simulink model "SPPMSM_DynoLoadTorque_sfun"  (R2022b)
settings: Solver=FixedStepDiscrete  StartTime=0.0  StopTime=SimTime  FixedStep=Ts_Model  RelTol=1e-3
undefined symbols (not defined in the file): theta_m_0
libraries: MapleSim_v142IE_1000 x1, MapleSim_v142IE_200 x1, MapleSim_v142IE_400 x1
settings Model: Creator=BEDNASA  LastModifiedBy=HENRIE2
settings SolverCC: AlgebraicLoopSolver=TrustRegion
settings DebuggingCC: UnconnectedInputMsg=warning  UnconnectedOutputMsg=warning  UnconnectedLineMsg=warning  SFMachineParentedDataDiag=warning
settings ModelReferenceCC: EnableRefExpFcnMdlSchedulingChecks=on
settings RTWCC: CustomInclude="\"C:\\Users\\BEDNASA\\Desktop\\SPPMSM\\SPPMSM\\SinglePhaseSimArch_alpha\\tools\\FMIKit-Simulink-2.8\\include\" \"C:\\Users\\BEDNASA\\Desktop\\VA_PSCSimulationArchitecture (2)\\VA_PSCSimulationArchitecture\\tools\\FMIKit-Simulink-2.7\\include\" \"C:\\Users\\BEDNASA\\Desktop\\SPPMSM\\SPPMSM\\MBD_SPM_SimArch\\tools\\include\" \"C:\\Users\\BEDNASA\\Desktop\\SPPMSM\\SPPMSM\\MBD_SPM_SimArch\\tools\\FMIKit\\FMIKit-Simulink-2.9\\include\" \"C:\\Data\\MBD_SPM_SimArch\\tools\\FMIKit\\FMIKit-Simulink-2.9\\include\" \"C:\\Users\\BEDNASA\\Desktop\\Projects\\MBD_SPM_SimArch_v02beta\\MBD_SPM_SimArch\\tools\\FMIKit\\FMIKit-Simulink-2.9\\include\" \"C:\\Data\\Szymon_Projects\\MBD_SPM_SimArch\\tools\\FMIKit\\FMIKit-Simulink-2.9\\include\" \"C:\\Data\\MBD_SPM_SimArch_TEST3\\tools\\FMIKit\\FMIKit-Simulink-2.9\\include\""  CustomSource="\"C:\\Users\\BEDNASA\\Desktop\\SPPMSM\\SPPMSM\\SinglePhaseSimArch_alpha\\tools\\FMIKit-Simulink-2.8\\src\\FMU.cpp\" \"C:\\Users\\BEDNASA\\Desktop\\SPPMSM\\SPPMSM\\SinglePhaseSimArch_alpha\\tools\\FMIKit-Simulink-2.8\\src\\FMU1.cpp\" \"C:\\Users\\BEDNASA\\Desktop\\SPPMSM\\SPPMSM\\SinglePhaseSimArch_alpha\\tools\\FMIKit-Simulink-2.8\\src\\FMU2.cpp\" \"C:\\Users\\BEDNASA\\Desktop\\VA_PSCSimulationArchitecture (2)\\VA_PSCSimulationArchitecture\\tools\\FMIKit-Simulink-2.7\\src\\FMU.cpp\" \"C:\\Users\\BEDNASA\\Desktop\\VA_PSCSimulationArchitecture (2)\\VA_PSCSimulationArchitecture\\tools\\FMIKit-Simulink-2.7\\src\\FMU1.cpp\" \"C:\\Users\\BEDNASA\\Desktop\\VA_PSCSimulationArchitecture (2)\\VA_PSCSimulationArchitecture\\tools\\FMIKit-Simulink-2.7\\src\\FMU2.cpp\" \"C:\\Users\\BEDNASA\\Desktop\\SPPMSM\\SPPMSM\\MBD_SPM_SimArch\\tools\\src\\FMU.cpp\" \"C:\\Users\\BEDNASA\\Desktop\\SPPMSM\\SPPMSM\\MBD_SPM_SimArch\\tools\\src\\FMU1.cpp\" \"C:\\Users\\BEDNASA\\Desktop\\SPPMSM\\SPPMSM\\MBD_SPM_SimArch\\tools\\src\\FMU2.cpp\" \"C:\\Users\\BEDNASA\\Desktop\\SPPMSM\\SPPMSM\\MBD_SPM_SimArch\\tools\\FMIKit\\FMIKit-Simulink-2.9\\src\\FMU.cpp\" \"C:\\Users\\BEDNASA\\Desktop\\SPPMSM\\SPPMSM\\MBD_SPM_SimArch\\tools\\FMIKit\\FMIKit-Simulink-2.9\\src\\FMU1.cpp\" \"C:\\Users\\BEDNASA\\Desktop\\SPPMSM\\SPPMSM\\MBD_SPM_SimArch\\tools\\FMIKit\\FMIKit-Simulink-2.9\\src\\FMU2.cpp\" \"C:\\Data\\MBD_SPM_SimArch\\tools\\FMIKit\\FMIKit-Simulink-2.9\\src\\FMU.cpp\" \"C:\\Data\\MBD_SPM_SimArch\\tools\\FMIKit\\FMIKit-Simulink-2.9\\src\\FMU1.cpp\" \"C:\\Data\\MBD_SPM_SimArch\\tools\\FMIKit\\FMIKit-Simulink-2.9\\src\\FMU2.cpp\" \"C:\\Users\\BEDNASA\\Desktop\\Projects\\MBD_SPM_SimArch_v02beta\\MBD_SPM_SimArch\\tools\\FMIKit\\FMIKit-Simulink-2.9\\src\\FMU.cpp\" \"C:\\Users\\BEDNASA\\Desktop\\Projects\\MBD_SPM_SimArch_v02beta\\MBD_SPM_SimArch\\tools\\FMIKit\\FMIKit-Simulink-2.9\\src\\FMU1.cpp\" \"C:\\Users\\BEDNASA\\Desktop\\Projects\\MBD_SPM_SimArch_v02beta\\MBD_SPM_SimArch\\tools\\FMIKit\\FMIKit-Simulink-2.9\\src\\FMU2.cpp\" \"C:\\Data\\Szymon_Projects\\MBD_SPM_SimArch\\tools\\FMIKit\\FMIKit-Simulink-2.9\\src\\FMU.cpp\" \"C:\\Data\\Szymon_Projects\\MBD_SPM_SimArch\\tools\\FMIKit\\FMIKit-Simulink-2.9\\src\\FMU1.cpp\" \"C:\\Data\\Szymon_Projects\\MBD_SPM_SimArch\\tools\\FMIKit\\FMIKit-Simulink-2.9\\src\\FMU2.cpp\" \"C:\\Data\\MBD_SPM_SimArch_TEST3\\tools\\FMIKit\\FMIKit-Simulink-2.9\\src\\FMU.cpp\" \"C:\\Data\\MBD_SPM_SimArch_TEST3\\tools\\FMIKit\\FMIKit-Simulink-2.9\\src\\FMU1.cpp\" \"C:\\Data\\MBD_SPM_SimArch_TEST3\\tools\\FMIKit\\FMIKit-Simulink-2.9\\src\\FMU2.cpp\""  CustomLibrary="\"C:\\Program Files\\Microsoft SDKs\\Windows\\v6.0A\\Lib\\x64\\ShLwApi.Lib\""

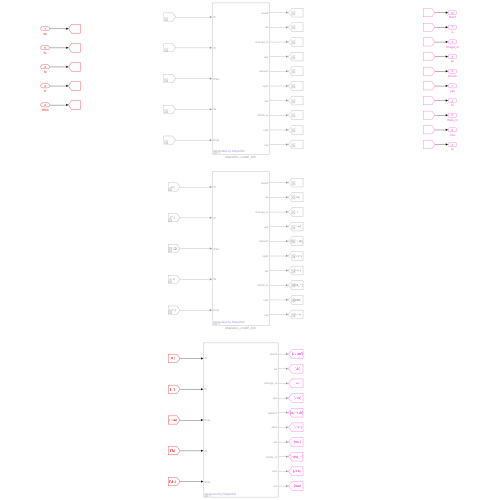
[thumbnail: Simulink's stored preview of the top-level diagram]
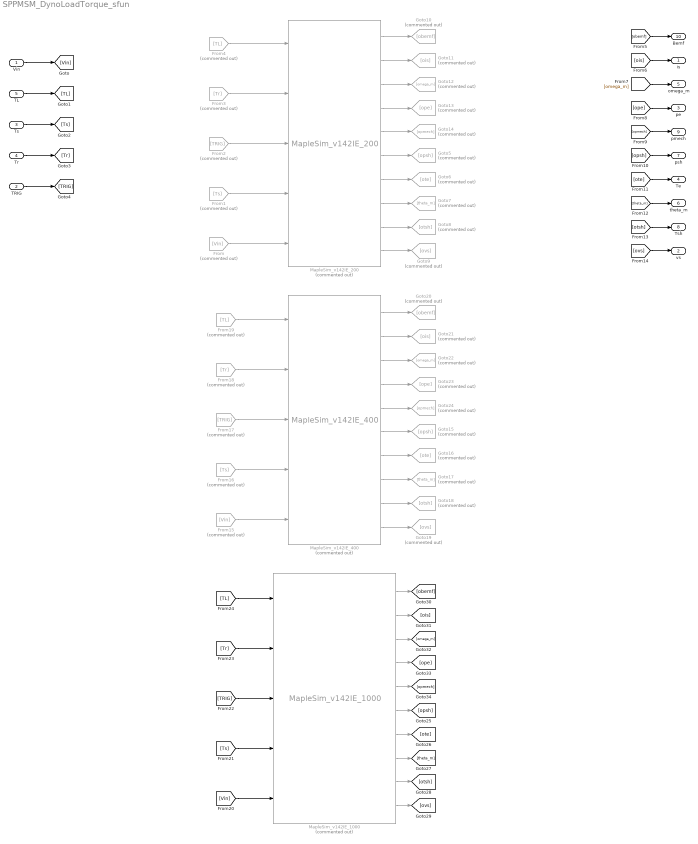
== system SPPMSM_DynoLoadTorque_sfun ==
  Vin : Inport
  TRIG : Inport  Port=2
  Ts : Inport  Port=3
  Tr : Inport  Port=4
  TL : Inport  Port=5
  From : From  Commented=on  GotoTag=Vin
  From1 : From  Commented=on  GotoTag=Ts
  From15 : From  Commented=on  GotoTag=Vin
  From16 : From  Commented=on  GotoTag=Ts
  From17 : From  Commented=on  GotoTag=TRIG
  From18 : From  Commented=on  GotoTag=Tr
  From19 : From  Commented=on  GotoTag=TL
  From2 : From  Commented=on  GotoTag=TRIG
  From3 : From  Commented=on  GotoTag=Tr
  From4 : From  Commented=on  GotoTag=TL
  Goto10 : Goto  Commented=on  GotoTag=obemf
  Goto11 : Goto  Commented=on  GotoTag=ois
  Goto12 : Goto  Commented=on  GotoTag=omega_m
  Goto13 : Goto  Commented=on  GotoTag=ope
  Goto14 : Goto  Commented=on  GotoTag=opmech
  Goto15 : Goto  Commented=on  GotoTag=opsh
  Goto16 : Goto  Commented=on  GotoTag=ote
  Goto17 : Goto  Commented=on  GotoTag=theta_m
  Goto18 : Goto  Commented=on  GotoTag=otsh
  Goto19 : Goto  Commented=on  GotoTag=ovs
  Goto20 : Goto  Commented=on  GotoTag=obemf
  Goto21 : Goto  Commented=on  GotoTag=ois
  Goto22 : Goto  Commented=on  GotoTag=omega_m
  Goto23 : Goto  Commented=on  GotoTag=ope
  Goto24 : Goto  Commented=on  GotoTag=opmech
  Goto5 : Goto  Commented=on  GotoTag=opsh
  Goto6 : Goto  Commented=on  GotoTag=ote
  Goto7 : Goto  Commented=on  GotoTag=theta_m
  Goto8 : Goto  Commented=on  GotoTag=otsh
  Goto9 : Goto  Commented=on  GotoTag=ovs
  MapleSim_v142IE_1000 : MapleSim_v142IE_1000/MapleSim_v142IE_1000  Description=Subsystem: MapleSim_v142IE_1000  Commented=on  ic=[theta_m_0, 0.]  Par1=B  Par2=PM_Flux_f01  Par3=StatorFluxMax  Par4=Jrotor  Par5=Jadd  Par6=Ls0  Par7=Lsmin  Par8=NPP  Par9=Rs0  Par10=22.  Par11=Trp  Par12=22.  Par13=alpha_s  Par14=d_magnet  Par15=-1.  Par16=0.  Par17=.5  Par18=1.  Par19=1.  Par20=1.  Par21=1.  Par22=.1e-4  Par23=.1e-4  Par24=.8  Par25=293.15  Par26=293.15  Par27=theta_m_0  MinStep=1/40
  MapleSim_v142IE_200 : MapleSim_v142IE_200/MapleSim_v142IE_200  Description=Subsystem: MapleSim_v142IE_200  Commented=on  ic=[theta_m_0, 0.]  Par1=B  Par2=PM_Flux_f01  Par3=StatorFluxMax  Par4=Jrotor  Par5=Jadd  Par6=Ls0  Par7=Lsmin  Par8=NPP  Par9=Rs0  Par10=PM_Temperature_Ref  Par11=Trp  Par12=PM_Temperature_Ref  Par13=alpha_s  Par14=d_magnet  Par15=-1.  Par16=0.  Par17=.5  Par18=1.  Par19=1.  Par20=1.  Par21=1.  Par22=.1e-4  Par23=.1e-4  Par24=.8  Par25=293.15  Par26=293.15  Par27=theta_m_0  MinStep=1/40
      link override sfn: Parameters=ExtData,MinStep
  MapleSim_v142IE_400 : MapleSim_v142IE_400/MapleSim_v142IE_400  Description=Subsystem: MapleSim_v142IE_400  Commented=on  ic=[theta_m_0, 0.]  Par1=B  Par2=PM_Flux_f01  Par3=StatorFluxMax  Par4=Jrotor  Par5=Jadd  Par6=Ls0  Par7=Lsmin  Par8=NPP  Par9=Rs0  Par10=PM_Temperature_Ref  Par11=Trp  Par12=PM_Temperature_Ref  Par13=alpha_s  Par14=d_magnet  Par15=-1.  Par16=0.  Par17=.5  Par18=1.  Par19=1.  Par20=1.  Par21=1.  Par22=.1e-4  Par23=.1e-4  Par24=.8  Par25=293.15  Par26=293.15  Par27=theta_m_0  MinStep=1/40
  is : Outport
  vs : Outport  Port=2
  pe : Outport  Port=3
  Te : Outport  Port=4
  omega_m : Outport  Port=5
  theta_m : Outport  Port=6
  psh : Outport  Port=7
  Tsh : Outport  Port=8
  pmech : Outport  Port=9
  Bemf : Outport  Port=10
  wires:
  Vin/1 -> [Vin]
  TL/1 -> [TL]
  Ts/1 -> [Ts]
  Tr/1 -> [Tr]
  TRIG/1 -> [TRIG]
  From/1 -> MapleSim_v142IE_200/5
  From1/1 -> MapleSim_v142IE_200/4
  From2/1 -> MapleSim_v142IE_200/3
  From3/1 -> MapleSim_v142IE_200/2
  From4/1 -> MapleSim_v142IE_200/1
  [obemf] -> Bemf/1
  [ois] -> is/1
  [omega_m] -> omega_m/1
  [opmech] -> pmech/1
  [ope] -> pe/1
  [opsh] -> psh/1
  [ote] -> Te/1
  [theta_m] -> theta_m/1
  [otsh] -> Tsh/1
  [ovs] -> vs/1
  From19/1 -> MapleSim_v142IE_400/1
  From18/1 -> MapleSim_v142IE_400/2
  From17/1 -> MapleSim_v142IE_400/3
  From16/1 -> MapleSim_v142IE_400/4
  From15/1 -> MapleSim_v142IE_400/5
  MapleSim_v142IE_400/3 -> Goto22/1
  MapleSim_v142IE_400/2 -> Goto21/1
  MapleSim_v142IE_400/1 -> Goto20/1
  MapleSim_v142IE_400/4 -> Goto23/1
  MapleSim_v142IE_400/5 -> Goto24/1
  MapleSim_v142IE_400/6 -> Goto15/1
  MapleSim_v142IE_400/7 -> Goto16/1
  MapleSim_v142IE_400/8 -> Goto17/1
  MapleSim_v142IE_400/9 -> Goto18/1
  MapleSim_v142IE_400/10 -> Goto19/1
  MapleSim_v142IE_200/6 -> Goto5/1
  MapleSim_v142IE_200/4 -> Goto13/1
  MapleSim_v142IE_200/10 -> Goto9/1
  MapleSim_v142IE_200/5 -> Goto14/1
  MapleSim_v142IE_200/9 -> Goto8/1
  MapleSim_v142IE_200/2 -> Goto11/1
  MapleSim_v142IE_200/8 -> Goto7/1
  MapleSim_v142IE_200/3 -> Goto12/1
  MapleSim_v142IE_200/1 -> Goto10/1
  MapleSim_v142IE_200/7 -> Goto6/1
  MapleSim_v142IE_1000/5 -> [opmech]
  MapleSim_v142IE_1000/6 -> [opsh]
  MapleSim_v142IE_1000/4 -> [ope]
  MapleSim_v142IE_1000/8 -> [theta_m]
  MapleSim_v142IE_1000/10 -> [ovs]
  MapleSim_v142IE_1000/7 -> [ote]
  MapleSim_v142IE_1000/9 -> [otsh]
  MapleSim_v142IE_1000/2 -> [ois]
  MapleSim_v142IE_1000/3 -> [omega_m]
  [Vin] -> MapleSim_v142IE_1000/5
  [TRIG] -> MapleSim_v142IE_1000/3
  [TL] -> MapleSim_v142IE_1000/1
  [Tr] -> MapleSim_v142IE_1000/2
  MapleSim_v142IE_1000/1 -> [obemf]
  [Ts] -> MapleSim_v142IE_1000/4
